simulink library "RF"  (Simulink 4.00)
values from neighbouring files (symbols this model uses):
  A = rms(interp1(f,MX,fb))    [fftbandamp.m]    (also in logfft.m = fftamp(samples, fs, f, varargin{:})/vpp; plotfft.m = fftamp(samples, fs, f, varargin{:})*2/vpp)
  P = sinc((1575.42 - f)/10.23).^2./10.23    [L1PSD.m]    (also in fftphase.m = interp1(f,PX,f0))
undefined symbols (not defined in the file or in its folder): adb, B, CA_ID, fs, j, m, N, p, Phi, Range, Rice_K, Rice_Seed, Rice_Sigma, tau_delay, z
libraries: RF x133, dspcmplx x47, com_sour x8, dspelmat x8, com_chan x4, dspbdsp x3, dspswit x3, simulink_extras x2, com_filt x2
(part 4 of 5)

== system RF/GPS Blocks/Low IF Receiver with  QBP Sigma-Delta ==
  note: Low IF with Quadrature Bandpass Sigma Delta
  RF In : Inport  Port=1
  4th Order Quadrature Bandpass Sigma-Delta with Mismatch : RF/A//D Blocks/4th Order Quadrature Bandpass Sigma-Delta with Mismatch  NTF_Poles=[0.67605+0.28003i 0.84752+0.10317i 0.67224+0.52633i 0.87023-0.35538i]  NTF_Zeros=[0.94544+0.3258i 0.92388+0.38268i 0.8989+0.43815i 0.92388-0.38268i]  STF_Zeros=[0.79335-0.60876i 0.13053+0.99144i 0.87023-0.35538i]  STF_Gain=0.95  ErrorStd=1  fs=80E6
  5th Order Complex Demodulation and Decimation : RF/A//D Blocks/5th Order Complex Demodulation and Decimation  fs=80E6  fIF=5E6  N=40
  Complex  Image-Reject  Filter with Mismatch : RF/Filters/Complex  Image-Reject  Filter with Mismatch  fc=250  f0=100  ErrorStd=1
  Join : dspcmplx/Join
  Join1 : dspcmplx/Join
  Non-Ideal Mixer : RF/Circuit Models/Non-Ideal Mixer  Gain1=0  IIP2=-500  IIP3=-500  fmax=1200  V1dB=1.5  AWGNVRMS=1E-12  SeedAWGN=1  Fseed=2  f0=1000  N0=1.147E-7  fm=10E3  numtaps=100
  Non-Ideal Mixer1 : RF/Circuit Models/Non-Ideal Mixer  Gain1=0  IIP2=-500  IIP3=-500  fmax=1200  V1dB=1.5  AWGNVRMS=1E-12  SeedAWGN=1  Fseed=2  f0=1000  N0=1.147E-7  fm=10E3  numtaps=100
  Non-Ideal  LNA : RF/Circuit Models/Non-Ideal  LNA  Gain1=0  IIP2=30  IIP3=20  AWGNVRMS=1E-3  fmax=3E9  V1dB=-4  SeedAWGN=123  FSeed=2  f0=1000  N0=1.147E-7  fm=10E3  numtaps=100
  Quadrature Oscillator : RF/Circuit Models/Quadrature Oscillator  PhiE=0  AE=0  Phi=0  A=1  f0=1573.42E6
  RF Filter1 : RF/Filters/RF Filter  Q=5  f0=1575.42E6  n=1  Gi=1
  Data Out : Outport  Port=1
  wires:
  Non-Ideal Mixer/1 -> Join/1
  Non-Ideal Mixer1/1 -> Join/2
  4th Order Quadrature Bandpass Sigma-Delta with Mismatch/1 -> 5th Order Complex Demodulation and Decimation/1
  Join1/1 -> Data Out/1
  5th Order Complex Demodulation and Decimation/1 -> Join1/1
  5th Order Complex Demodulation and Decimation/2 -> Join1/2
  RF Filter1/1 -> Non-Ideal  LNA/1
  RF In/1 -> RF Filter1/1
  Non-Ideal  LNA/1 -> Non-Ideal Mixer1/1, Non-Ideal Mixer/2
  Quadrature Oscillator/1 -> Non-Ideal Mixer/1
  Quadrature Oscillator/2 -> Non-Ideal Mixer1/2
  Join/1 -> Complex  Image-Reject  Filter with Mismatch/1
  Complex  Image-Reject  Filter with Mismatch/1 -> 4th Order Quadrature Bandpass Sigma-Delta with Mismatch/1

== system RF/GPS Blocks/Navigation Data ==
  "Data, 50Hz" : Subsystem  mask(Random integer generator){mul=2, seed=Seed}
      mask prompts: mul "M-ary number:"
      mask help: Generate integers randomly distributed in range [0, M-1], where M is the M-ary number.
      mask init:
      | [x,y]=srcsicon(4);
      settings: RTWFcnNameOpts=Auto  RTWFileNameOpts=Auto
      mask Help: This block generates an integer number in the range [0 M-1], where M is the M-ary number. The probability of the appearance for each number is equal.
      mask Display: plot(0,0,100,100,x,y);disp('Random int')
  Zero-Order Hold : ZeroOrderHold  SampleTime=1/50
  Out1 : Outport  Port=1  InitialOutput=0
  wires:
  "Data, 50Hz"/1(out_1) -> Zero-Order Hold/1
  Zero-Order Hold/1 -> Out1/1

== system RF/Miscellaneous/Clocked  Integrator ==
  In1 : Inport  Port=1
  Trigger : TriggerPort  TriggerType=rising  OutputDataType=auto
  Sum : Sum  Inputs=|++  SaturateOnIntegerOverflow=on
  Unit Delay : UnitDelay  Orientation=left  X0=0  SampleTime=-1
  Out1 : Outport  Port=1
  wires:
  In1/1 -> Sum/1
  Sum/1 -> Out1/1, Unit Delay/1
  Unit Delay/1 -> Sum/2

== system RF/Miscellaneous/Clocked Delaying Integrator ==
  In1 : Inport  Port=1
  Trigger : TriggerPort  TriggerType=rising  OutputDataType=auto
  Sum : Sum  Inputs=|++  SaturateOnIntegerOverflow=on
  Unit Delay : UnitDelay  X0=0  SampleTime=-1
  Out1 : Outport  Port=1
  wires:
  In1/1 -> Sum/1
  Unit Delay/1 -> Sum/2, Out1/1
  Sum/1 -> Unit Delay/1

== system RF/Miscellaneous/Inverse dB ==
  in : Inport  Port=1
  Gain : Gain  Gain=1/g  Multiplication=Element-wise(K.*u)  SaturateOnIntegerOverflow=on
  Math Function : Math  Operator=10^u  OutputSignalType=auto
  out : Outport  Port=1  InitialOutput=0
  wires:
  Math Function/1 -> out/1
  Gain/1 -> Math Function/1
  in/1 -> Gain/1

== system RF/Miscellaneous/Linear ==
  In1 : Inport  Port=1
  Constant : Constant  Value=Offset
  Gain : Gain  Gain=Gain  Multiplication=Element-wise(K.*u)  SaturateOnIntegerOverflow=on
  Sum1 : Sum  Inputs=|++  SaturateOnIntegerOverflow=on
  Out1 : Outport  Port=1
  wires:
  In1/1 -> Gain/1
  Sum1/1 -> Out1/1
  Constant/1 -> Sum1/2
  Gain/1 -> Sum1/1

== system RF/Miscellaneous/Maximum Magnitude Switch ==
  In : Inport  Port=1
  In1 : Inport  Port=2
  Abs : Abs  SaturateOnIntegerOverflow=on
  Abs1 : Abs  SaturateOnIntegerOverflow=on
  Sum : Sum  Inputs=+-  SaturateOnIntegerOverflow=on
  Switch : Switch  Threshold=0
  Out1 : Outport  Port=1  InitialOutput=0
  wires:
  Abs1/1 -> Sum/2
  In1/1 -> Switch/3, Abs1/1
  In/1 -> Switch/1, Abs/1
  Switch/1 -> Out1/1
  Sum/1 -> Switch/2
  Abs/1 -> Sum/1

== system RF/Miscellaneous/Minimum Magnitude Switch ==
  In : Inport  Port=1
  In1 : Inport  Port=2
  Abs : Abs  SaturateOnIntegerOverflow=on
  Abs1 : Abs  SaturateOnIntegerOverflow=on
  Sum : Sum  Inputs=-+  SaturateOnIntegerOverflow=on
  Switch : Switch  Threshold=0
  Out1 : Outport  Port=1  InitialOutput=0
  wires:
  Abs1/1 -> Sum/2
  In1/1 -> Switch/3, Abs1/1
  In/1 -> Switch/1, Abs/1
  Switch/1 -> Out1/1
  Sum/1 -> Switch/2
  Abs/1 -> Sum/1

== system RF/Miscellaneous/N-Sample Switch w/Reset ==
  In1 : Inport  Port=1
  In2 : Inport  Port=2
  Enable : EnablePort  StatesWhenEnabling=reset
  N-Sample Switch : dspswit/N-Sample Switch  N=N  Ts=Ts
  Out1 : Outport  Port=1  InitialOutput=0
  wires:
  In2/1 -> N-Sample Switch/2
  N-Sample Switch/1 -> Out1/1
  In1/1 -> N-Sample Switch/1

== system RF/Miscellaneous/PFD ==
  A : Inport  Port=1
  B : Inport  Port=2
  Constant : Constant  Value=1
  D Flip-Flop : simulink_extras/Flip Flops/D Flip-Flop
  D Flip-Flop1 : simulink_extras/Flip Flops/D Flip-Flop
  Logical Operator : Logic  Orientation=left  Operator=NAND  Inputs=2
  Terminator : Terminator
  Terminator1 : Terminator
  QA : Outport  Port=1
  QB : Outport  Port=2
  wires:
  D Flip-Flop1/1 -> QB/1, Logical Operator/2
  D Flip-Flop/1 -> QA/1, Logical Operator/1
  B/1 -> D Flip-Flop1/2
  A/1 -> D Flip-Flop/2
  D Flip-Flop/2 -> Terminator1/1
  D Flip-Flop1/2 -> Terminator/1
  Logical Operator/1 -> D Flip-Flop1/3, D Flip-Flop/3
  Constant/1 -> D Flip-Flop1/1, D Flip-Flop/1

== system RF/Model Nonidealities/Amplitude and Phase Error ==
  In1 : Inport  Port=1
  Amplitude Error : Gain  Gain=A  Multiplication=Element-wise(K.*u)  SaturateOnIntegerOverflow=on
  Phase Error : TransportDelay  DelayTime=Phi  InitialInput=0  BufferSize=1024  PadeOrder=0
  Out1 : Outport  Port=1  InitialOutput=0
  wires:
  In1/1 -> Amplitude Error/1
  Phase Error/1 -> Out1/1
  Amplitude Error/1 -> Phase Error/1

== system RF/Model Nonidealities/Compression ==
  In1 : Inport  Port=1
  Trigonometric Function1 : Trigonometry  Operator=tanh  OutputSignalType=auto
  dB Gain : dspelmat/dB Gain  dB=-Adjust  intype=Amplitude
  dB Gain1 : dspelmat/dB Gain  dB=Adjust  intype=Amplitude
  Out1 : Outport  Port=1  InitialOutput=0
  wires:
  In1/1 -> dB Gain/1
  dB Gain/1 -> Trigonometric Function1/1
  dB Gain1/1 -> Out1/1
  Trigonometric Function1/1 -> dB Gain1/1

== system RF/Model Nonidealities/Flicker Noise ==
  Discrete Filter : DiscreteFilter  Numerator=1  Denominator=a  SampleTime=ts  Realization=auto
  Gain : Gain  Gain=g  Multiplication=Element-wise(K.*u)  SaturateOnIntegerOverflow=on
  Random Number : RandomNumber  Mean=0  Variance=1  Seed=Seed  SampleTime=0
  Out1 : Outport  Port=1  InitialOutput=0
  wires:
  Gain/1 -> Discrete Filter/1
  Discrete Filter/1 -> Out1/1
  Random Number/1 -> Gain/1

== system RF/Model Nonidealities/Nonlinear TF ==
  In1 : Inport  Orientation=down  Port=1
  Constant Exponent : dspelmat/Constant Exponent  k=2
  Constant Exponent1 : dspelmat/Constant Exponent  k=3
  Sum : Sum  Inputs=+--  SaturateOnIntegerOverflow=on
  dB Gain : dspelmat/dB Gain  dB=Gain2  intype=Amplitude
  dB Gain1 : dspelmat/dB Gain  dB=Gain3  intype=Amplitude
  dB Gain3 : dspelmat/dB Gain  dB=Gain1  intype=Amplitude
  Out1 : Outport  Port=1  InitialOutput=0
  wires:
  Constant Exponent1/1 -> dB Gain1/1
  Constant Exponent/1 -> dB Gain/1
  dB Gain1/1 -> Sum/3
  dB Gain/1 -> Sum/2
  dB Gain3/1 -> Constant Exponent1/1, Constant Exponent/1, Sum/1
  Sum/1 -> Out1/1
  In1/1 -> dB Gain3/1

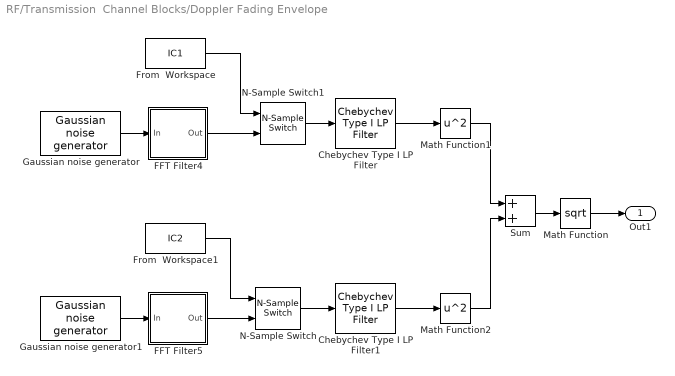
== system RF/Transmission  Channel Blocks/Doppler Fading Envelope ==
  Chebychev Type I LP Filter : RF/Filters/Chebychev Type I LP Filter  w0=100*2*pi  n=8  ripple=0.5
  Chebychev Type I LP Filter1 : RF/Filters/Chebychev Type I LP Filter  w0=100*2*pi  n=8  ripple=0.5
  FFT Filter4 : Subsystem  mask(FFT Filter){N=N, H=H, ts=ts}
      mask prompts: N "FFT size"; H "Filter Values"; ts "Sample time:"
      mask help: FFT based filtering;
      settings: RTWFcnNameOpts=Auto  RTWFileNameOpts=Auto
      mask Display: disp('FFT Filter');
  FFT Filter5 : Subsystem  mask(FFT Filter){N=N, H=H, ts=ts}
      mask prompts: N "FFT size"; H "Filter Values"; ts "Sample time:"
      mask help: FFT based filtering;
      settings: RTWFcnNameOpts=Auto  RTWFileNameOpts=Auto
      mask Display: disp('FFT Filter');
  From  Workspace : FromWorkspace  VariableName=IC1  SampleTime=-1  OutputAfterFinalValue=Extrapolation
  From  Workspace1 : FromWorkspace  VariableName=IC2  SampleTime=-1  OutputAfterFinalValue=Extrapolation
  Gaussian noise generator : com_sour/Gaussian noise generator  m=0  d=NVar  s=100
  Gaussian noise generator1 : com_sour/Gaussian noise generator  m=0  d=NVar  s=412
  Math Function : Math  Operator=sqrt  OutputSignalType=auto
  Math Function1 : Math  Operator=square  OutputSignalType=auto
  Math Function2 : Math  Operator=square  OutputSignalType=auto
  N-Sample Switch : dspswit/N-Sample Switch  N=2*N  Ts=ts
  N-Sample Switch1 : dspswit/N-Sample Switch  N=2*N  Ts=ts
  Sum : Sum  Inputs=++  SaturateOnIntegerOverflow=on
  Out1 : Outport  Port=1  InitialOutput=0
  wires:
  From  Workspace1/1 -> N-Sample Switch/1
  From  Workspace/1 -> N-Sample Switch1/1
  Sum/1 -> Math Function/1
  FFT Filter4/1(Out) -> N-Sample Switch1/2
  Gaussian noise generator/1 -> FFT Filter4/1(In)
  N-Sample Switch1/1 -> Chebychev Type I LP Filter/1
  FFT Filter5/1(Out) -> N-Sample Switch/2
  Gaussian noise generator1/1 -> FFT Filter5/1(In)
  N-Sample Switch/1 -> Chebychev Type I LP Filter1/1
  Chebychev Type I LP Filter1/1 -> Math Function2/1
  Chebychev Type I LP Filter/1 -> Math Function1/1
  Math Function/1 -> Out1/1
  Math Function2/1 -> Sum/2
  Math Function1/1 -> Sum/1

== system RF/Transmission  Channel Blocks/Doppler Fading with User Defined Filter ==
  note: Doppler Fading
  Baseband Doppler Filter : com_filt/Complex filter  num=Num  den=Denom  ts=ts
  Baseband Doppler Filter1 : com_filt/Complex filter  num=Num  den=Denom  ts=ts
  Gaussian noise generator : com_sour/Gaussian noise generator  m=0  d=NVar  s=Seed(1)
  Gaussian noise generator1 : com_sour/Gaussian noise generator  m=0  d=NVar  s=Seed(2)
  Gaussian noise generator2 : com_sour/Gaussian noise generator  m=0  d=NVar  s=Seed(3)
  Gaussian noise generator3 : com_sour/Gaussian noise generator  m=0  d=NVar  s=Seed(4)
  Join : dspcmplx/Join
  Join1 : dspcmplx/Join
  Magnitude Squared : dspcmplx/Magnitude Squared
  Magnitude Squared1 : dspcmplx/Magnitude Squared
  Math Function : Math  Operator=sqrt  OutputSignalType=auto
  Sum : Sum  Inputs=++  SaturateOnIntegerOverflow=on
  Out1 : Outport  Port=1  InitialOutput=0
  wires:
  Join1/1 -> Baseband Doppler Filter1/1
  Gaussian noise generator/1 -> Join/1
  Gaussian noise generator1/1 -> Join/2
  Gaussian noise generator2/1 -> Join1/1
  Gaussian noise generator3/1 -> Join1/2
  Join/1 -> Baseband Doppler Filter/1
  Baseband Doppler Filter/1 -> Magnitude Squared/1
  Baseband Doppler Filter1/1 -> Magnitude Squared1/1
  Magnitude Squared/1 -> Sum/1
  Magnitude Squared1/1 -> Sum/2
  Math Function/1 -> Out1/1
  Sum/1 -> Math Function/1

== system RF/Transmission  Channel Blocks/Doppler and  Multi-path Fading ==
  In : Inport  Port=1
  Doppler Fading Envelope : RF/Transmission  Channel Blocks/Doppler Fading Envelope  fm=20  N=1024  NVar=1
  Doppler Fading Envelope1 : RF/Transmission  Channel Blocks/Doppler Fading Envelope  fm=20  N=1024  NVar=1
  Doppler Fading Envelope2 : RF/Transmission  Channel Blocks/Doppler Fading Envelope  fm=20  N=1024  NVar=1
  Product1 : Product  Inputs=2  Multiplication=Element-wise(.*)  SaturateOnIntegerOverflow=on
  Product2 : Product  Inputs=2  Multiplication=Element-wise(.*)  SaturateOnIntegerOverflow=on
  Product3 : Product  Inputs=2  Multiplication=Element-wise(.*)  SaturateOnIntegerOverflow=on
  Sum : Sum  Inputs=++++  SaturateOnIntegerOverflow=on
  Transport Delay : TransportDelay  DelayTime=2*DelaySpread / 3  InitialInput=0  BufferSize=1024  PadeOrder=0
  Transport Delay1 : TransportDelay  DelayTime=DelaySpread  InitialInput=0  BufferSize=1024  PadeOrder=0
  Transport Delay2 : TransportDelay  DelayTime=DelaySpread / 3  InitialInput=0  BufferSize=1024  PadeOrder=0
  Out : Outport  Port=1  InitialOutput=0
  wires:
  Transport Delay2/1 -> Product3/2
  Doppler Fading Envelope/1 -> Product3/1
  Transport Delay/1 -> Product2/2
  Doppler Fading Envelope1/1 -> Product2/1
  Transport Delay1/1 -> Product1/2
  Doppler Fading Envelope2/1 -> Product1/1
  In/1 -> Transport Delay2/1, Transport Delay/1, Transport Delay1/1, Sum/4
  Product3/1 -> Sum/1
  Product1/1 -> Sum/3
  Product2/1 -> Sum/2
  Sum/1 -> Out/1

== system RF/Transmission  Channel Blocks/Exponential Path Loss and Log-Normal Shadowing ==
  note: Exponential Path Loss and Log-Normal Shadowing
  In : Inport  Port=1
  Constant : Constant  Value=d
  Constant2 : Constant  Value=p0
  Gain1 : Gain  Gain=1/d0  Multiplication=Element-wise(K.*u)  SaturateOnIntegerOverflow=on
  Inverse dB : RF/Miscellaneous/Inverse dB  intype=Amplitude
  Product : Product  Inputs=2  Multiplication=Element-wise(.*)  SaturateOnIntegerOverflow=on
  Random Number : RandomNumber  Mean=0  Variance=Sigma_P  Seed=0  SampleTime=0
  Sum : Sum  Inputs=++-  SaturateOnIntegerOverflow=on
  dB : dspelmat/dB  intype=Amplitude
  Out : Outport  Port=1  InitialOutput=0
  wires:
  Random Number/1 -> Sum/1
  Constant2/1 -> Sum/2
  dB/1 -> Sum/3
  Gain1/1 -> dB/1
  Sum/1 -> Inverse dB/1
  Constant/1 -> Gain1/1
  Product/1 -> Out/1
  Inverse dB/1 -> Product/2
  In/1 -> Product/1

== system RF/Transmission  Channel Blocks/Impulse Noise ==
  note: Impulse Noise
  Comparator : RF/Circuit Models/Comparator  L_Out=0  H_Out=1  Bound=1-P_Impulse
  Product : Product  Inputs=2  Multiplication=Element-wise(.*)  SaturateOnIntegerOverflow=on
  Random Number : RandomNumber  Mean=Amp_Mean  Variance=Amp_Var  Seed=0  SampleTime=-1
  Transfer Fcn : TransferFcn  Numerator=Num  Denominator=Denom  Realization=auto  AbsoluteTolerance=auto
  Uniform Random Number : UniformRandomNumber  Minimum=0  Maximum=1  Seed=0  SampleTime=-1
  Zero-Order Hold : ZeroOrderHold  SampleTime=T_Impulse
  Out1 : Outport  Port=1  InitialOutput=0
  wires:
  Product/1 -> Out1/1
  Random Number/1 -> Product/2
  Comparator/1 -> Transfer Fcn/1
  Zero-Order Hold/1 -> Comparator/1
  Uniform Random Number/1 -> Zero-Order Hold/1
  Transfer Fcn/1 -> Product/1

== system RF/Transmission  Channel Blocks/Out-of-Band  Interference ==
  Chebychev Type I Band Stop Filter : RF/Filters/Chebychev Type I Band Stop Filter  w1=2*pi*(fo-fbw/2)  w2=2*pi*(fo+fbw/2)  order=Order  ripple=Ripple
  Gaussian noise generator : com_sour/Gaussian noise generator  m=0  d=AWGNVRMS^2  s=AWGNSeed
  Sine Wave : Sin  Amplitude=Amplitudes  Frequency=Frequencies  Phase=Phases  SampleTime=0
  Sum : Sum  Inputs=1  SaturateOnIntegerOverflow=on
  Sum1 : Sum  Inputs=++  SaturateOnIntegerOverflow=on
  Out : Outport  Port=1  InitialOutput=0
  wires:
  Sum1/1 -> Out/1
  Sine Wave/1 -> Sum/1
  Sum/1 -> Sum1/2
  Chebychev Type I Band Stop Filter/1 -> Sum1/1
  Gaussian noise generator/1 -> Chebychev Type I Band Stop Filter/1

== system RF/A/D Blocks/Fourth Order Sigma Delta/Comparator ==
  In : Inport  Port=1
  Relay : Relay  OnSwitchValue=Bound  OffSwitchValue=Bound  OnOutputValue=H_Out  OffOutputValue=L_Out
  Out : Outport  Port=1  InitialOutput=0
  wires:
  Relay/1 -> Out/1
  In/1 -> Relay/1

== system RF/A/D Blocks/Fourth Order Sigma Delta with Mismatch/Comparator ==
  In : Inport  Port=1
  Relay : Relay  OnSwitchValue=Bound  OffSwitchValue=Bound  OnOutputValue=H_Out  OffOutputValue=L_Out
  Out : Outport  Port=1  InitialOutput=0
  wires:
  In/1 -> Relay/1
  Relay/1 -> Out/1

== system RF/A/D Blocks/Second Order Simple  Lowpass  Sigma-Delta/Comparator ==
  In : Inport  Port=1
  Relay : Relay  OnSwitchValue=Bound  OffSwitchValue=Bound  OnOutputValue=H_Out  OffOutputValue=L_Out
  Out : Outport  Port=1  InitialOutput=0
  wires:
  Relay/1 -> Out/1
  In/1 -> Relay/1

== system RF/A/D Blocks/Simple Lowpass  Sigma-Delta/Comparator ==
  In : Inport  Port=1
  Relay : Relay  OnSwitchValue=Bound  OffSwitchValue=Bound  OnOutputValue=H_Out  OffOutputValue=L_Out
  Out : Outport  Port=1  InitialOutput=0
  wires:
  Relay/1 -> Out/1
  In/1 -> Relay/1

== system RF/A/D Blocks/Simple Quadrature BandPass Sigma-Delta/Complex Resonator ==
  In1 : Inport  Port=1
  Complex Gain : RF/Complex Blocks/Complex Gain  G=-1
  Complex Unit Delay : RF/Complex Blocks/Complex Unit Delay  icr=1  ici=1  ts=ts
  Complex Unit Delay1 : RF/Complex Blocks/Complex Unit Delay  icr=1  ici=1  ts=ts
  Complex Sum1 : dspcmplx/Complex Sum  Inputs=++
  Out1 : Outport  Port=1  InitialOutput=0
  wires:
  Complex Gain/1 -> Out1/1, Complex Sum1/1
  Complex Unit Delay1/1 -> Complex Gain/1
  Complex Unit Delay/1 -> Complex Unit Delay1/1
  In1/1 -> Complex Sum1/2
  Complex Sum1/1 -> Complex Unit Delay/1

== system RF/GPS Blocks/C/A Code, 1.023MHz/PN1 ==
  note: PRN Sequence Generator
  1-step delay1 : Subsystem  mask(Multi-step delay){n=1, ts=1/1.023E6, ini=1}
      mask prompts: n "Delay steps (integer):"; ts "Sample time (sec):"; ini "Initial output:"
      mask help: Output is K-step delay of the input signal.
      mask init:
      | if length(ts)<2, ts=[ts 0];end;
      settings: RTWFcnNameOpts=Auto  RTWFileNameOpts=Auto
      mask Help: This block holds the input signal for K steps and then outputs the signal. The delay step cannot be changed during the simulation.
      mask Display: disp('-k\nz   ')
  1-step delay100 : Subsystem  mask(Multi-step delay){n=1, ts=1/1.023E6, ini=1}
      mask prompts: n "Delay steps (integer):"; ts "Sample time (sec):"; ini "Initial output:"
      mask help: Output is K-step delay of the input signal.
      mask init:
      | if length(ts)<2, ts=[ts 0];end;
      settings: RTWFcnNameOpts=Auto  RTWFileNameOpts=Auto
      mask Help: This block holds the input signal for K steps and then outputs the signal. The delay step cannot be changed during the simulation.
      mask Display: disp('-k\nz   ')
  1-step delay2 : Subsystem  mask(Multi-step delay){n=1, ts=1/1.023E6, ini=1}
      mask prompts: n "Delay steps (integer):"; ts "Sample time (sec):"; ini "Initial output:"
      mask help: Output is K-step delay of the input signal.
      mask init:
      | if length(ts)<2, ts=[ts 0];end;
      settings: RTWFcnNameOpts=Auto  RTWFileNameOpts=Auto
      mask Help: This block holds the input signal for K steps and then outputs the signal. The delay step cannot be changed during the simulation.
      mask Display: disp('-k\nz   ')
  1-step delay3 : Subsystem  mask(Multi-step delay){n=1, ts=1/1.023E6, ini=1}
      mask prompts: n "Delay steps (integer):"; ts "Sample time (sec):"; ini "Initial output:"
      mask help: Output is K-step delay of the input signal.
      mask init:
      | if length(ts)<2, ts=[ts 0];end;
      settings: RTWFcnNameOpts=Auto  RTWFileNameOpts=Auto
      mask Help: This block holds the input signal for K steps and then outputs the signal. The delay step cannot be changed during the simulation.
      mask Display: disp('-k\nz   ')
  1-step delay4 : Subsystem  mask(Multi-step delay){n=1, ts=1/1.023E6, ini=1}
      mask prompts: n "Delay steps (integer):"; ts "Sample time (sec):"; ini "Initial output:"
      mask help: Output is K-step delay of the input signal.
      mask init:
      | if length(ts)<2, ts=[ts 0];end;
      settings: RTWFcnNameOpts=Auto  RTWFileNameOpts=Auto
      mask Help: This block holds the input signal for K steps and then outputs the signal. The delay step cannot be changed during the simulation.
      mask Display: disp('-k\nz   ')
  1-step delay5 : Subsystem  mask(Multi-step delay){n=1, ts=1/1.023E6, ini=1}
      mask prompts: n "Delay steps (integer):"; ts "Sample time (sec):"; ini "Initial output:"
      mask help: Output is K-step delay of the input signal.
      mask init:
      | if length(ts)<2, ts=[ts 0];end;
      settings: RTWFcnNameOpts=Auto  RTWFileNameOpts=Auto
      mask Help: This block holds the input signal for K steps and then outputs the signal. The delay step cannot be changed during the simulation.
      mask Display: disp('-k\nz   ')
  1-step delay6 : Subsystem  mask(Multi-step delay){n=1, ts=1/1.023E6, ini=1}
      mask prompts: n "Delay steps (integer):"; ts "Sample time (sec):"; ini "Initial output:"
      mask help: Output is K-step delay of the input signal.
      mask init:
      | if length(ts)<2, ts=[ts 0];end;
      settings: RTWFcnNameOpts=Auto  RTWFileNameOpts=Auto
      mask Help: This block holds the input signal for K steps and then outputs the signal. The delay step cannot be changed during the simulation.
      mask Display: disp('-k\nz   ')
  1-step delay7 : Subsystem  mask(Multi-step delay){n=1, ts=1/1.023E6, ini=1}
      mask prompts: n "Delay steps (integer):"; ts "Sample time (sec):"; ini "Initial output:"
      mask help: Output is K-step delay of the input signal.
      mask init:
      | if length(ts)<2, ts=[ts 0];end;
      settings: RTWFcnNameOpts=Auto  RTWFileNameOpts=Auto
      mask Help: This block holds the input signal for K steps and then outputs the signal. The delay step cannot be changed during the simulation.
      mask Display: disp('-k\nz   ')
  1-step delay8 : Subsystem  mask(Multi-step delay){n=1, ts=1/1.023E6, ini=1}
      mask prompts: n "Delay steps (integer):"; ts "Sample time (sec):"; ini "Initial output:"
      mask help: Output is K-step delay of the input signal.
      mask init:
      | if length(ts)<2, ts=[ts 0];end;
      settings: RTWFcnNameOpts=Auto  RTWFileNameOpts=Auto
      mask Help: This block holds the input signal for K steps and then outputs the signal. The delay step cannot be changed during the simulation.
      mask Display: disp('-k\nz   ')
  1-step delay9 : Subsystem  mask(Multi-step delay){n=1, ts=1/1.023E6, ini=1}
      mask prompts: n "Delay steps (integer):"; ts "Sample time (sec):"; ini "Initial output:"
      mask help: Output is K-step delay of the input signal.
      mask init:
      | if length(ts)<2, ts=[ts 0];end;
      settings: RTWFcnNameOpts=Auto  RTWFileNameOpts=Auto
      mask Help: This block holds the input signal for K steps and then outputs the signal. The delay step cannot be changed during the simulation.
      mask Display: disp('-k\nz   ')
  Adder : Logic  Orientation=left  Operator=XOR  Inputs=2
  Tap10 : Outport  Port=1  InitialOutput=0
  wires:
  1-step delay100/1(out_1) -> Tap10/1, Adder/1
  1-step delay1/1(out_1) -> 1-step delay2/1(in_1)
  1-step delay2/1(out_1) -> 1-step delay3/1(in_1)
  1-step delay4/1(out_1) -> 1-step delay5/1(in_1)
  1-step delay5/1(out_1) -> 1-step delay6/1(in_1)
  1-step delay6/1(out_1) -> 1-step delay7/1(in_1)
  1-step delay7/1(out_1) -> 1-step delay8/1(in_1)
  1-step delay8/1(out_1) -> 1-step delay9/1(in_1)
  1-step delay9/1(out_1) -> 1-step delay100/1(in_1)
  Adder/1 -> 1-step delay1/1(in_1)
  1-step delay3/1(out_1) -> 1-step delay4/1(in_1), Adder/2

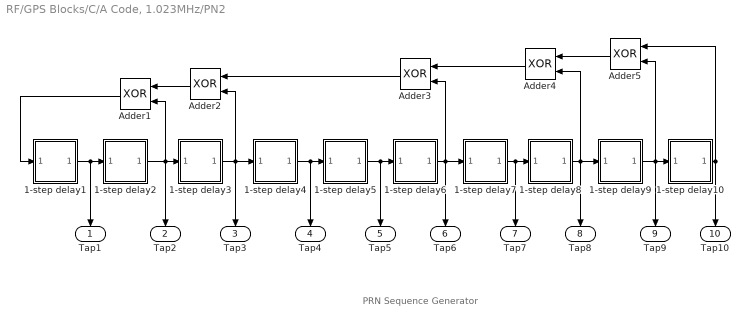
== system RF/GPS Blocks/C/A Code, 1.023MHz/PN2 ==
  note: PRN Sequence Generator
  1-step delay1 : Subsystem  mask(Multi-step delay){n=1, ts=1/1.023E6, ini=1}
      mask prompts: n "Delay steps (integer):"; ts "Sample time (sec):"; ini "Initial output:"
      mask help: Output is K-step delay of the input signal.
      mask init:
      | if length(ts)<2, ts=[ts 0];end;
      settings: RTWFcnNameOpts=Auto  RTWFileNameOpts=Auto
      mask Help: This block holds the input signal for K steps and then outputs the signal. The delay step cannot be changed during the simulation.
      mask Display: disp('-k\nz   ')
  1-step delay10 : Subsystem  mask(Multi-step delay){n=1, ts=1/1.023E6, ini=1}
      mask prompts: n "Delay steps (integer):"; ts "Sample time (sec):"; ini "Initial output:"
      mask help: Output is K-step delay of the input signal.
      mask init:
      | if length(ts)<2, ts=[ts 0];end;
      settings: RTWFcnNameOpts=Auto  RTWFileNameOpts=Auto
      mask Help: This block holds the input signal for K steps and then outputs the signal. The delay step cannot be changed during the simulation.
      mask Display: disp('-k\nz   ')
  1-step delay2 : Subsystem  mask(Multi-step delay){n=1, ts=1/1.023E6, ini=1}
      mask prompts: n "Delay steps (integer):"; ts "Sample time (sec):"; ini "Initial output:"
      mask help: Output is K-step delay of the input signal.
      mask init:
      | if length(ts)<2, ts=[ts 0];end;
      settings: RTWFcnNameOpts=Auto  RTWFileNameOpts=Auto
      mask Help: This block holds the input signal for K steps and then outputs the signal. The delay step cannot be changed during the simulation.
      mask Display: disp('-k\nz   ')
  1-step delay3 : Subsystem  mask(Multi-step delay){n=1, ts=1/1.023E6, ini=1}
      mask prompts: n "Delay steps (integer):"; ts "Sample time (sec):"; ini "Initial output:"
      mask help: Output is K-step delay of the input signal.
      mask init:
      | if length(ts)<2, ts=[ts 0];end;
      settings: RTWFcnNameOpts=Auto  RTWFileNameOpts=Auto
      mask Help: This block holds the input signal for K steps and then outputs the signal. The delay step cannot be changed during the simulation.
      mask Display: disp('-k\nz   ')
  1-step delay4 : Subsystem  mask(Multi-step delay){n=1, ts=1/1.023E6, ini=1}
      mask prompts: n "Delay steps (integer):"; ts "Sample time (sec):"; ini "Initial output:"
      mask help: Output is K-step delay of the input signal.
      mask init:
      | if length(ts)<2, ts=[ts 0];end;
      settings: RTWFcnNameOpts=Auto  RTWFileNameOpts=Auto
      mask Help: This block holds the input signal for K steps and then outputs the signal. The delay step cannot be changed during the simulation.
      mask Display: disp('-k\nz   ')
  1-step delay5 : Subsystem  mask(Multi-step delay){n=1, ts=1/1.023E6, ini=1}
      mask prompts: n "Delay steps (integer):"; ts "Sample time (sec):"; ini "Initial output:"
      mask help: Output is K-step delay of the input signal.
      mask init:
      | if length(ts)<2, ts=[ts 0];end;
      settings: RTWFcnNameOpts=Auto  RTWFileNameOpts=Auto
      mask Help: This block holds the input signal for K steps and then outputs the signal. The delay step cannot be changed during the simulation.
      mask Display: disp('-k\nz   ')
  1-step delay6 : Subsystem  mask(Multi-step delay){n=1, ts=1/1.023E6, ini=1}
      mask prompts: n "Delay steps (integer):"; ts "Sample time (sec):"; ini "Initial output:"
      mask help: Output is K-step delay of the input signal.
      mask init:
      | if length(ts)<2, ts=[ts 0];end;
      settings: RTWFcnNameOpts=Auto  RTWFileNameOpts=Auto
      mask Help: This block holds the input signal for K steps and then outputs the signal. The delay step cannot be changed during the simulation.
      mask Display: disp('-k\nz   ')
  1-step delay7 : Subsystem  mask(Multi-step delay){n=1, ts=1/1.023E6, ini=1}
      mask prompts: n "Delay steps (integer):"; ts "Sample time (sec):"; ini "Initial output:"
      mask help: Output is K-step delay of the input signal.
      mask init:
      | if length(ts)<2, ts=[ts 0];end;
      settings: RTWFcnNameOpts=Auto  RTWFileNameOpts=Auto
      mask Help: This block holds the input signal for K steps and then outputs the signal. The delay step cannot be changed during the simulation.
      mask Display: disp('-k\nz   ')
  1-step delay8 : Subsystem  mask(Multi-step delay){n=1, ts=1/1.023E6, ini=1}
      mask prompts: n "Delay steps (integer):"; ts "Sample time (sec):"; ini "Initial output:"
      mask help: Output is K-step delay of the input signal.
      mask init:
      | if length(ts)<2, ts=[ts 0];end;
      settings: RTWFcnNameOpts=Auto  RTWFileNameOpts=Auto
      mask Help: This block holds the input signal for K steps and then outputs the signal. The delay step cannot be changed during the simulation.
      mask Display: disp('-k\nz   ')
  1-step delay9 : Subsystem  mask(Multi-step delay){n=1, ts=1/1.023E6, ini=1}
      mask prompts: n "Delay steps (integer):"; ts "Sample time (sec):"; ini "Initial output:"
      mask help: Output is K-step delay of the input signal.
      mask init:
      | if length(ts)<2, ts=[ts 0];end;
      settings: RTWFcnNameOpts=Auto  RTWFileNameOpts=Auto
      mask Help: This block holds the input signal for K steps and then outputs the signal. The delay step cannot be changed during the simulation.
      mask Display: disp('-k\nz   ')
  Adder{1..5} (5 alike) : Logic  Orientation=left  Operator=XOR  Inputs=2
  Tap1 : Outport  Orientation=down  Port=1  InitialOutput=0
  Tap2 : Outport  Orientation=down  Port=2  InitialOutput=0
  Tap3 : Outport  Orientation=down  Port=3  InitialOutput=0
  Tap4 : Outport  Orientation=down  Port=4  InitialOutput=0
  Tap5 : Outport  Orientation=down  Port=5  InitialOutput=0
  Tap6 : Outport  Orientation=down  Port=6  InitialOutput=0
  Tap7 : Outport  Orientation=down  Port=7  InitialOutput=0
  Tap8 : Outport  Orientation=down  Port=8  InitialOutput=0
  Tap9 : Outport  Orientation=down  Port=9  InitialOutput=0
  Tap10 : Outport  Orientation=down  Port=10  InitialOutput=0
  wires:
  1-step delay10/1(out_1) -> Tap10/1, Adder5/1
  1-step delay7/1(out_1) -> Tap7/1, 1-step delay8/1(in_1)
  1-step delay5/1(out_1) -> Tap5/1, 1-step delay6/1(in_1)
  1-step delay4/1(out_1) -> Tap4/1, 1-step delay5/1(in_1)
  1-step delay1/1(out_1) -> Tap1/1, 1-step delay2/1(in_1)
  1-step delay2/1(out_1) -> Tap2/1, 1-step delay3/1(in_1), Adder1/2
  Adder2/1 -> Adder1/1
  1-step delay3/1(out_1) -> Tap3/1, Adder2/2, 1-step delay4/1(in_1)
  1-step delay6/1(out_1) -> Tap6/1, 1-step delay7/1(in_1), Adder3/2
  Adder3/1 -> Adder2/1
  Adder4/1 -> Adder3/1
  1-step delay8/1(out_1) -> Tap8/1, Adder4/2, 1-step delay9/1(in_1)
  Adder5/1 -> Adder4/1
  1-step delay9/1(out_1) -> Tap9/1, 1-step delay10/1(in_1), Adder5/2
  Adder1/1 -> 1-step delay1/1(in_1)

== system RF/GPS Blocks/GPS Channel/AWGN channel ==
  in_1 : Inport  Port=1
  Gaussian noise generator1 : Subsystem  mask(Gaussian noise generator){m=m, d=d, s=s}
      mask prompts: m "Mean value:"; d "Variance (vector or matrix):"; s "Initial seed:"
      mask help: Generate Gaussian distributed noise with given mean and variance value.
      mask init:
      | [m,d,s]=gwnoise(m,d,s);
      settings: RTWFcnNameOpts=Auto  RTWFileNameOpts=Auto
      mask Help: When the mean value and seed are vectors, the output of this block is a vector. The length of the vector is the same as the length of the mean value vector or the length of the seed. When the variance entry is a vector, the variance is a diagonal matrix.
      mask Display:
      | plot(0,0,100,100,[95 5 10 10 10 (100-15)*[0:1/30:1]+10],[75 75 75 70 95 rand(1,31)*20+75]);
      | disp('Gaussian')
  Sum : Sum  Inputs=++  SaturateOnIntegerOverflow=on
  out_1 : Outport  Port=1  InitialOutput=0
  wires:
  Gaussian noise generator1/1(out_1) -> Sum/2
  Sum/1 -> out_1/1
  in_1/1 -> Sum/1

== system RF/GPS Blocks/GPS Transmitter/BPSK mod, 1575MHz1 ==
  in_1 : Inport  Port=1
  MPSK map : Subsystem  mask(MPSK map){td=td}
      mask prompts: td "M-ary number (input integer in range [0, M-1]):"
      mask help: Map input digital signal to analog phase shift.
      mask init:
      | pi2=2*pi;Sft=pi2/@1;
      settings: RTWFcnNameOpts=Auto  RTWFileNameOpts=Auto
      mask Help: This block maps the input digital signal to the analog signal, which is ready for the PM modulation. The input are integers in the range [0, M-1], where M is the M-ary number. You can view the MPSK constellation using the MODMAP function.
      mask Display: disp('MPSK\nmap')
  PM passband : Subsystem  mask(Passband PM){Fc=Fc, Ph=Ph, td=td, ts=ts}
      mask prompts: Fc "Carrier frequency (Hz):"; Ph "Initial phase (rad):"; td "Symbol interval (sec, Use inf for analog case):"; ts "Sample Time"
      mask help: Modulate the input signal using PM method.
      mask init:
      | Fc=Fc*2*pi;if isinf(td),td=realmax;end;
      settings: RTWFcnNameOpts=Auto  RTWFileNameOpts=Auto
      mask Help: The PM block causes the change of the carrier signal depending on the input signal voltage.
      mask Display:
      | plot(0,0,100,100,[4.5*[0:10]+5 50 50 50 50+4.5*[0:.15:10]],[10*sin([0:10]*pi/5)+85 85 99 75 85+10*[sin([0:.15:10]*pi*2+cumsum(sin([0:.15:10]*pi/5))/2)]]);
      | disp('PM')
  out_1 : Outport  Port=1  InitialOutput=0
  wires:
  in_1/1 -> MPSK map/1(in_1)
  PM passband/1(out_1) -> out_1/1
  MPSK map/1(out_1) -> PM passband/1(in_1)

== system RF/GPS Blocks/GPS Transmitter/BPSK mod, 1575MHz2 ==
  in_1 : Inport  Port=1
  MPSK map : Subsystem  mask(MPSK map){td=td}
      mask prompts: td "M-ary number (input integer in range [0, M-1]):"
      mask help: Map input digital signal to analog phase shift.
      mask init:
      | pi2=2*pi;Sft=pi2/@1;
      settings: RTWFcnNameOpts=Auto  RTWFileNameOpts=Auto
      mask Help: This block maps the input digital signal to the analog signal, which is ready for the PM modulation. The input are integers in the range [0, M-1], where M is the M-ary number. You can view the MPSK constellation using the MODMAP function.
      mask Display: disp('MPSK\nmap')
  PM passband : Subsystem  mask(Passband PM){Fc=Fc, Ph=Ph, td=td, ts=ts}
      mask prompts: Fc "Carrier frequency (Hz):"; Ph "Initial phase (rad):"; td "Symbol interval (sec, Use inf for analog case):"; ts "Sample Time"
      mask help: Modulate the input signal using PM method.
      mask init:
      | Fc=Fc*2*pi;if isinf(td),td=realmax;end;
      settings: RTWFcnNameOpts=Auto  RTWFileNameOpts=Auto
      mask Help: The PM block causes the change of the carrier signal depending on the input signal voltage.
      mask Display:
      | plot(0,0,100,100,[4.5*[0:10]+5 50 50 50 50+4.5*[0:.15:10]],[10*sin([0:10]*pi/5)+85 85 99 75 85+10*[sin([0:.15:10]*pi*2+cumsum(sin([0:.15:10]*pi/5))/2)]]);
      | disp('PM')
  out_1 : Outport  Port=1  InitialOutput=0
  wires:
  in_1/1 -> MPSK map/1(in_1)
  PM passband/1(out_1) -> out_1/1
  MPSK map/1(out_1) -> PM passband/1(in_1)

== system RF/GPS Blocks/GPS Transmitter/P Code, 10.23MHz ==
  "P Code, 10.23MHz" : Subsystem  mask(Random integer generator){mul=2, seed=P_Seed}
      mask prompts: mul "M-ary number:"
      mask help: Generate integers randomly distributed in range [0, M-1], where M is the M-ary number.
      mask init:
      | [x,y]=srcsicon(4);
      settings: RTWFcnNameOpts=Auto  RTWFileNameOpts=Auto
      mask Help: This block generates an integer number in the range [0 M-1], where M is the M-ary number. The probability of the appearance for each number is equal.
      mask Display: plot(0,0,100,100,x,y);disp('Random int')
  Zero-Order Hold : ZeroOrderHold  SampleTime=1/10.23E6
  Out1 : Outport  Port=1  InitialOutput=0
  wires:
  "P Code, 10.23MHz"/1(out_1) -> Zero-Order Hold/1
  Zero-Order Hold/1 -> Out1/1

== system RF/GPS Blocks/Navigation Data/Data, 50Hz ==
  Uniform number : S-Function  FunctionName=srandint  Parameters=seed,mul  PortCounts=[]  SFunctionModules=''
  out_1 : Outport  Port=1  InitialOutput=0
  wires:
  Uniform number/1 -> out_1/1

== system RF/Transmission  Channel Blocks/Doppler Fading Envelope/FFT Filter4 ==
  In : Inport  Port=1
  Buffer : Subsystem  mask(Buffer){N=N, V=0, Ts=ts, ic=0}
      mask prompts: N "Buffer size:"; V "Buffer overlap:"; Ts "Input sample time:"; ic "Initial  condition:"
      mask help: Convert scalar samples to a vector output at a lower sample rate.
      settings: RTWFcnNameOpts=Auto  RTWFileNameOpts=Auto
      mask Help: web(dspbhelp);
      mask Display: plot(0,0,100,100,[12 28 28 32 28 28],[92 92 94 92 90 92],[32 36 36 40 36 36],[92 92 94 92 90 92],[24 24 28],[92 92 92],[40 44 44 48 44 44],[92 92 94 92 90 92],[52 48 52 52 56 52 52],[92 92 92 94 92 90 92],[56 64 64 57 64 71],[92 92 69 76 69 76],[48 80 80 48 48],[64 64 12 12 64],[56 72],[56 56],[56 72],[48 48],[56 72],[40 40],[56 72],[32 32],[56 72],[24 24])
  Complex Multiply1 : Subsystem  mask(Complex Multiply){}
      mask help: Compute element-wise multiplication of complex inputs.
      mask init:
      | [x,y]=cplxico2;
      settings: RTWFcnNameOpts=Auto  RTWFileNameOpts=Auto
      mask Help: web(dspbhelp);
      mask Display: plot(x,y);disp(' x')
  Filter Response : Subsystem  mask(Complex Constant){val=H}
      mask prompts: val "Constant complex value:"
      mask help: Generate a constant complex output value.
      mask init:
      | C=[real(val(:)).',imag(val(:)).'];
      | [x,y]=cplxico2;
      settings: RTWFcnNameOpts=Auto  RTWFileNameOpts=Auto
      mask Help: web(dspbhelp);
      mask Display:
      | plot(x,y);
      | text(15,50,&1,'h','l','v','m');
  Partial Unbuffer : Subsystem  mask(Partial Unbuffer){N=N, N1=1, N2=N, num_chans=1, Ts=ts*N}
      mask prompts: N "Buffer size:"; N1 "First output index:"; N2 "Last output index:"; num_chans "Number of channels"; Ts "Input sample time:"
      mask help: Convert selected portion of a vector to scalar samples output at a higher sample rate.
      mask init:
      | elements=repmat(0:N:(num_chans-1)*N,N2-N1+1,1);
      | elements=elements(:)';
      | elements=elements + repmat(N1:N2,1,num_chans);
      settings: RTWFcnNameOpts=Auto  RTWFileNameOpts=Auto
      mask Help: web(dspbhelp);
      mask Display: plot(0,0,100,100,[62 68 68 72 68 68],[24 24 26 24 22 24],[36 36 56 49 56 49],[32 24 24 16 24 32],[20 52 52 20 20],[88 88 36 36 88],[28 44],[80 80],[28 44],[72 72],[28 44],[64 64],[28 44],[56 56],[28 44],[48 48],[72 76 76 80 76 76],[24 24 26 24 22 24],[80 84 84 88 84 84],[24 24 26 24 22 24],[],[],[],[],[88 88 92],[24 24 24])
  Real FFT : Subsystem  mask(Real FFT){}
      mask help: Fast Fourier transform of a real vector.
      mask init:
      | [x,y]=cplxico2(1,[]);
      settings: RTWFcnNameOpts=Auto  RTWFileNameOpts=Auto
      mask Help: web(dspbhelp);
      mask Display: plot(x,y);disp('  FFT ')
  Real IFFT : Subsystem  mask(Real IFFT){}
      mask help: Inverse fast Fourier transform of a complex vector with conjugate symmetry.
      mask init:
      | [x,y]=cplxico2([],1);
      settings: RTWFcnNameOpts=Auto  RTWFileNameOpts=Auto
      mask Help: web(dspbhelp);
      mask Display: plot(x,y);disp('  IFFT')
  Out : Outport  Port=1  InitialOutput=0
  wires:
  Partial Unbuffer/1(out_1) -> Out/1
  Real IFFT/1(out_1) -> Partial Unbuffer/1(in_1)
  Buffer/1(Outport) -> Real FFT/1(in_1)
  Complex Multiply1/1(Complex Multiply Result) -> Real IFFT/1(in_1)
  Filter Response/1(Out1) -> Complex Multiply1/2(Complex input 2)
  Real FFT/1(out_1) -> Complex Multiply1/1(Complex input 1)
  In/1 -> Buffer/1(in_1)

== system RF/Transmission  Channel Blocks/Doppler Fading Envelope/FFT Filter5 ==
  In : Inport  Port=1
  Buffer : Subsystem  mask(Buffer){N=N, V=0, Ts=ts, ic=0}
      mask prompts: N "Buffer size:"; V "Buffer overlap:"; Ts "Input sample time:"; ic "Initial  condition:"
      mask help: Convert scalar samples to a vector output at a lower sample rate.
      settings: RTWFcnNameOpts=Auto  RTWFileNameOpts=Auto
      mask Help: web(dspbhelp);
      mask Display: plot(0,0,100,100,[12 28 28 32 28 28],[92 92 94 92 90 92],[32 36 36 40 36 36],[92 92 94 92 90 92],[24 24 28],[92 92 92],[40 44 44 48 44 44],[92 92 94 92 90 92],[52 48 52 52 56 52 52],[92 92 92 94 92 90 92],[56 64 64 57 64 71],[92 92 69 76 69 76],[48 80 80 48 48],[64 64 12 12 64],[56 72],[56 56],[56 72],[48 48],[56 72],[40 40],[56 72],[32 32],[56 72],[24 24])
  Complex Multiply1 : Subsystem  mask(Complex Multiply){}
      mask help: Compute element-wise multiplication of complex inputs.
      mask init:
      | [x,y]=cplxico2;
      settings: RTWFcnNameOpts=Auto  RTWFileNameOpts=Auto
      mask Help: web(dspbhelp);
      mask Display: plot(x,y);disp(' x')
  Filter Response : Subsystem  mask(Complex Constant){val=H}
      mask prompts: val "Constant complex value:"
      mask help: Generate a constant complex output value.
      mask init:
      | C=[real(val(:)).',imag(val(:)).'];
      | [x,y]=cplxico2;
      settings: RTWFcnNameOpts=Auto  RTWFileNameOpts=Auto
      mask Help: web(dspbhelp);
      mask Display:
      | plot(x,y);
      | text(15,50,&1,'h','l','v','m');
  Partial Unbuffer : Subsystem  mask(Partial Unbuffer){N=N, N1=1, N2=N, num_chans=1, Ts=ts*N}
      mask prompts: N "Buffer size:"; N1 "First output index:"; N2 "Last output index:"; num_chans "Number of channels"; Ts "Input sample time:"
      mask help: Convert selected portion of a vector to scalar samples output at a higher sample rate.
      mask init:
      | elements=repmat(0:N:(num_chans-1)*N,N2-N1+1,1);
      | elements=elements(:)';
      | elements=elements + repmat(N1:N2,1,num_chans);
      settings: RTWFcnNameOpts=Auto  RTWFileNameOpts=Auto
      mask Help: web(dspbhelp);
      mask Display: plot(0,0,100,100,[62 68 68 72 68 68],[24 24 26 24 22 24],[36 36 56 49 56 49],[32 24 24 16 24 32],[20 52 52 20 20],[88 88 36 36 88],[28 44],[80 80],[28 44],[72 72],[28 44],[64 64],[28 44],[56 56],[28 44],[48 48],[72 76 76 80 76 76],[24 24 26 24 22 24],[80 84 84 88 84 84],[24 24 26 24 22 24],[],[],[],[],[88 88 92],[24 24 24])
  Real FFT : Subsystem  mask(Real FFT){}
      mask help: Fast Fourier transform of a real vector.
      mask init:
      | [x,y]=cplxico2(1,[]);
      settings: RTWFcnNameOpts=Auto  RTWFileNameOpts=Auto
      mask Help: web(dspbhelp);
      mask Display: plot(x,y);disp('  FFT ')
  Real IFFT : Subsystem  mask(Real IFFT){}
      mask help: Inverse fast Fourier transform of a complex vector with conjugate symmetry.
      mask init:
      | [x,y]=cplxico2([],1);
      settings: RTWFcnNameOpts=Auto  RTWFileNameOpts=Auto
      mask Help: web(dspbhelp);
      mask Display: plot(x,y);disp('  IFFT')
  Out : Outport  Port=1  InitialOutput=0
  wires:
  Partial Unbuffer/1(out_1) -> Out/1
  Real IFFT/1(out_1) -> Partial Unbuffer/1(in_1)
  Buffer/1(Outport) -> Real FFT/1(in_1)
  Complex Multiply1/1(Complex Multiply Result) -> Real IFFT/1(in_1)
  Filter Response/1(Out1) -> Complex Multiply1/2(Complex input 2)
  Real FFT/1(out_1) -> Complex Multiply1/1(Complex input 1)
  In/1 -> Buffer/1(in_1)

== system RF/GPS Blocks/C/A Code, 1.023MHz/PN1/1-step delay1 ==
  in_1 : Inport  Port=1
  Constant : Constant  Value=ini
  Constant1 : Constant  Value=n*ts(1)+ts(2)
  Digital Clock : DigitalClock  SampleTime=ts
  K-step delay : DiscreteFilter  Numerator=[zeros(1,n), 1]  Denominator=1  SampleTime=ts  Realization=auto
  Relational Operator : RelationalOperator  Operator=>=
  Switch : Switch  Threshold=.1
  out_1 : Outport  Port=1  InitialOutput=0
  wires:
  Relational Operator/1 -> Switch/2
  Constant1/1 -> Relational Operator/2
  Digital Clock/1 -> Relational Operator/1
  Constant/1 -> Switch/3
  K-step delay/1 -> Switch/1
  in_1/1 -> K-step delay/1
  Switch/1 -> out_1/1

== system RF/GPS Blocks/C/A Code, 1.023MHz/PN1/1-step delay100 ==
  in_1 : Inport  Port=1
  Constant : Constant  Value=ini
  Constant1 : Constant  Value=n*ts(1)+ts(2)
  Digital Clock : DigitalClock  SampleTime=ts
  K-step delay : DiscreteFilter  Numerator=[zeros(1,n), 1]  Denominator=1  SampleTime=ts  Realization=auto
  Relational Operator : RelationalOperator  Operator=>=
  Switch : Switch  Threshold=.1
  out_1 : Outport  Port=1  InitialOutput=0
  wires:
  Relational Operator/1 -> Switch/2
  Constant1/1 -> Relational Operator/2
  Digital Clock/1 -> Relational Operator/1
  Constant/1 -> Switch/3
  K-step delay/1 -> Switch/1
  in_1/1 -> K-step delay/1
  Switch/1 -> out_1/1

== system RF/GPS Blocks/C/A Code, 1.023MHz/PN1/1-step delay2 ==
  in_1 : Inport  Port=1
  Constant : Constant  Value=ini
  Constant1 : Constant  Value=n*ts(1)+ts(2)
  Digital Clock : DigitalClock  SampleTime=ts
  K-step delay : DiscreteFilter  Numerator=[zeros(1,n), 1]  Denominator=1  SampleTime=ts  Realization=auto
  Relational Operator : RelationalOperator  Operator=>=
  Switch : Switch  Threshold=.1
  out_1 : Outport  Port=1  InitialOutput=0
  wires:
  Relational Operator/1 -> Switch/2
  Constant1/1 -> Relational Operator/2
  Digital Clock/1 -> Relational Operator/1
  Constant/1 -> Switch/3
  K-step delay/1 -> Switch/1
  in_1/1 -> K-step delay/1
  Switch/1 -> out_1/1

== system RF/GPS Blocks/C/A Code, 1.023MHz/PN1/1-step delay3 ==
  in_1 : Inport  Port=1
  Constant : Constant  Value=ini
  Constant1 : Constant  Value=n*ts(1)+ts(2)
  Digital Clock : DigitalClock  SampleTime=ts
  K-step delay : DiscreteFilter  Numerator=[zeros(1,n), 1]  Denominator=1  SampleTime=ts  Realization=auto
  Relational Operator : RelationalOperator  Operator=>=
  Switch : Switch  Threshold=.1
  out_1 : Outport  Port=1  InitialOutput=0
  wires:
  Relational Operator/1 -> Switch/2
  Constant1/1 -> Relational Operator/2
  Digital Clock/1 -> Relational Operator/1
  Constant/1 -> Switch/3
  K-step delay/1 -> Switch/1
  in_1/1 -> K-step delay/1
  Switch/1 -> out_1/1

== system RF/GPS Blocks/C/A Code, 1.023MHz/PN1/1-step delay4 ==
  in_1 : Inport  Port=1
  Constant : Constant  Value=ini
  Constant1 : Constant  Value=n*ts(1)+ts(2)
  Digital Clock : DigitalClock  SampleTime=ts
  K-step delay : DiscreteFilter  Numerator=[zeros(1,n), 1]  Denominator=1  SampleTime=ts  Realization=auto
  Relational Operator : RelationalOperator  Operator=>=
  Switch : Switch  Threshold=.1
  out_1 : Outport  Port=1  InitialOutput=0
  wires:
  Relational Operator/1 -> Switch/2
  Constant1/1 -> Relational Operator/2
  Digital Clock/1 -> Relational Operator/1
  Constant/1 -> Switch/3
  K-step delay/1 -> Switch/1
  in_1/1 -> K-step delay/1
  Switch/1 -> out_1/1

== system RF/GPS Blocks/C/A Code, 1.023MHz/PN1/1-step delay5 ==
  in_1 : Inport  Port=1
  Constant : Constant  Value=ini
  Constant1 : Constant  Value=n*ts(1)+ts(2)
  Digital Clock : DigitalClock  SampleTime=ts
  K-step delay : DiscreteFilter  Numerator=[zeros(1,n), 1]  Denominator=1  SampleTime=ts  Realization=auto
  Relational Operator : RelationalOperator  Operator=>=
  Switch : Switch  Threshold=.1
  out_1 : Outport  Port=1  InitialOutput=0
  wires:
  Relational Operator/1 -> Switch/2
  Constant1/1 -> Relational Operator/2
  Digital Clock/1 -> Relational Operator/1
  Constant/1 -> Switch/3
  K-step delay/1 -> Switch/1
  in_1/1 -> K-step delay/1
  Switch/1 -> out_1/1

== system RF/GPS Blocks/C/A Code, 1.023MHz/PN1/1-step delay6 ==
  in_1 : Inport  Port=1
  Constant : Constant  Value=ini
  Constant1 : Constant  Value=n*ts(1)+ts(2)
  Digital Clock : DigitalClock  SampleTime=ts
  K-step delay : DiscreteFilter  Numerator=[zeros(1,n), 1]  Denominator=1  SampleTime=ts  Realization=auto
  Relational Operator : RelationalOperator  Operator=>=
  Switch : Switch  Threshold=.1
  out_1 : Outport  Port=1  InitialOutput=0
  wires:
  Relational Operator/1 -> Switch/2
  Constant1/1 -> Relational Operator/2
  Digital Clock/1 -> Relational Operator/1
  Constant/1 -> Switch/3
  K-step delay/1 -> Switch/1
  in_1/1 -> K-step delay/1
  Switch/1 -> out_1/1

== system RF/GPS Blocks/C/A Code, 1.023MHz/PN1/1-step delay7 ==
  in_1 : Inport  Port=1
  Constant : Constant  Value=ini
  Constant1 : Constant  Value=n*ts(1)+ts(2)
  Digital Clock : DigitalClock  SampleTime=ts
  K-step delay : DiscreteFilter  Numerator=[zeros(1,n), 1]  Denominator=1  SampleTime=ts  Realization=auto
  Relational Operator : RelationalOperator  Operator=>=
  Switch : Switch  Threshold=.1
  out_1 : Outport  Port=1  InitialOutput=0
  wires:
  Relational Operator/1 -> Switch/2
  Constant1/1 -> Relational Operator/2
  Digital Clock/1 -> Relational Operator/1
  Constant/1 -> Switch/3
  K-step delay/1 -> Switch/1
  in_1/1 -> K-step delay/1
  Switch/1 -> out_1/1

== system RF/GPS Blocks/C/A Code, 1.023MHz/PN1/1-step delay8 ==
  in_1 : Inport  Port=1
  Constant : Constant  Value=ini
  Constant1 : Constant  Value=n*ts(1)+ts(2)
  Digital Clock : DigitalClock  SampleTime=ts
  K-step delay : DiscreteFilter  Numerator=[zeros(1,n), 1]  Denominator=1  SampleTime=ts  Realization=auto
  Relational Operator : RelationalOperator  Operator=>=
  Switch : Switch  Threshold=.1
  out_1 : Outport  Port=1  InitialOutput=0
  wires:
  Relational Operator/1 -> Switch/2
  Constant1/1 -> Relational Operator/2
  Digital Clock/1 -> Relational Operator/1
  Constant/1 -> Switch/3
  K-step delay/1 -> Switch/1
  in_1/1 -> K-step delay/1
  Switch/1 -> out_1/1
